simulink model "PID_differential_drive_robot"  (R2023b)
settings: Solver=VariableStepAuto  StartTime=0.0  StopTime=20  RelTol=1e-3
settings Model: Creator=patel  LastModifiedBy=patel

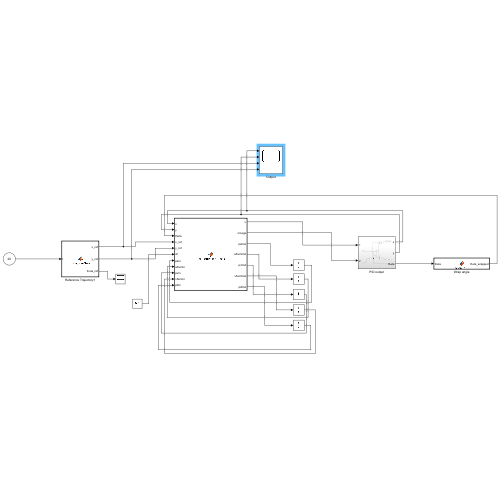
[thumbnail: Simulink's stored preview of the top-level diagram]
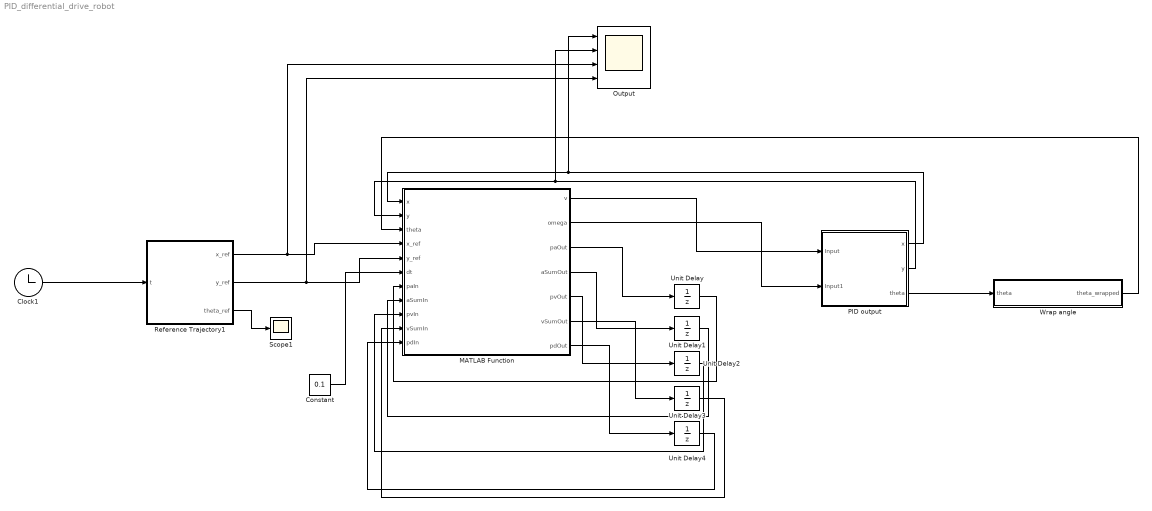
== system PID_differential_drive_robot ==
  Clock1 : Clock
      settings: Decimation=20
  Constant : Constant  Value=0.1
  MATLAB Function : MATLAB Function  TreatAsAtomicUnit=on
  Output : Scope  NumInputPorts=4
  PID output : Subsystem
  Reference Trajectory1 : MATLAB Function  TreatAsAtomicUnit=on
  Scope1 : Scope
  Unit Delay{,1..4} (5 alike) : UnitDelay  SampleTime=-1  HasFrameUpgradeWarning=on
  Wrap angle : MATLAB Function  TreatAsAtomicUnit=on
  wires:
  Clock1/1 -> Reference Trajectory1/1(t)
  Reference Trajectory1/1(x_ref) -> Output/3, MATLAB Function/4(x_ref)
  Reference Trajectory1/2(y_ref) -> Output/4, MATLAB Function/5(y_ref)
  Reference Trajectory1/3(theta_ref) -> Scope1/1
  MATLAB Function/1(v) -> PID output/1(Input)
  MATLAB Function/2(omega) -> PID output/2(Input1)
  PID output/3(theta) -> Wrap angle/1(theta)
  PID output/1(x) -> Output/1, MATLAB Function/1(x)
  PID output/2(y) -> Output/2, MATLAB Function/2(y)
  Wrap angle/1(theta_wrapped) -> MATLAB Function/3(theta)
  Constant/1 -> MATLAB Function/6(dt)
  MATLAB Function/3(paOut) -> Unit Delay/1
  Unit Delay/1 -> MATLAB Function/7(paIn)
  MATLAB Function/4(aSumOut) -> Unit Delay1/1
  Unit Delay1/1 -> MATLAB Function/8(aSumIn)
  MATLAB Function/5(pvOut) -> Unit Delay2/1
  Unit Delay2/1 -> MATLAB Function/9(pvIn)
  MATLAB Function/6(vSumOut) -> Unit Delay3/1
  Unit Delay3/1 -> MATLAB Function/10(vSumIn)
  MATLAB Function/7(pdOut) -> Unit Delay4/1
  Unit Delay4/1 -> MATLAB Function/11(pdIn)

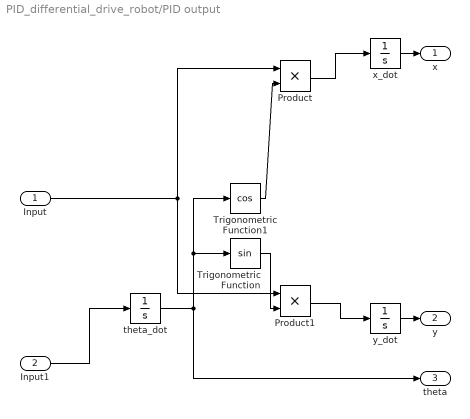
== system PID_differential_drive_robot/PID output ==
  Input : Inport
  Input1 : Inport  Port=2
  Product : Product
  Product1 : Product
  Trigonometric Function : Trigonometry
  Trigonometric Function1 : Trigonometry  Operator=cos
  theta_dot : Integrator
  x_dot : Integrator
  y_dot : Integrator
  x : Outport
  y : Outport  Port=2
  theta : Outport  Port=3
  wires:
  theta_dot/1 -> theta/1, Trigonometric Function1/1, Trigonometric Function/1
  Product/1 -> x_dot/1
  Input1/1 -> theta_dot/1
  Trigonometric Function1/1 -> Product/2
  Input/1 -> Product1/1, Product/1
  Trigonometric Function/1 -> Product1/2
  Product1/1 -> y_dot/1
  x_dot/1 -> x/1
  y_dot/1 -> y/1

== matlab function PID_differential_drive_robot/Wrap angle ==
  data: theta input; theta_wrapped output
function theta_wrapped = wrapToPi(theta)
    theta_wrapped = mod(theta + pi, 2*pi) - pi;
end

== matlab function PID_differential_drive_robot/MATLAB Function ==
  data: x input; v output; y input; theta input; x_ref input; y_ref input; dt input; paIn input; aSumIn input; pvIn input; vSumIn input; pdIn input; omega output; paOut output; aSumOut output; pvOut output; vSumOut output; pdOut output
function [v, omega, paOut, aSumOut, pvOut, vSumOut, pdOut] = pid_controller_block(x, y, theta, x_ref, y_ref, dt, paIn, aSumIn, pvIn, vSumIn, pdIn)
%#codegen
robotState = [x; y; theta];
targetPoint = [x_ref; y_ref];
[v, omega, paOut, aSumOut, pvOut, vSumOut, pdOut] = PIDController(robotState, targetPoint, dt, paIn, aSumIn, pvIn, vSumIn, pdIn);

    function [v, omega, prevAngleError, angleErrorSum, prevVError, vErrorSum, prevDistance] = PIDController(robotState, targetPoint, dt, prevAngleError, angleErrorSum, prevVError, vErrorSum, prevDistance)
    % Unpack robot state
    x = robotState(1);
    y = robotState(2);
    theta = robotState(3);

    x_target = targetPoint(1);
    y_target = targetPoint(2);

    % Desired forward velocity
    v_desired = 5.0;

    %% --- Angular control (omega) ---
    angle_to_target = atan2(y_target - y, x_target - x);
    angle_error = atan2(sin(angle_to_target - theta), cos(angle_to_target - theta));
    angle_error_deriv = (angle_error - prevAngleError) / dt;
    angleErrorSum = angleErrorSum + angle_error * dt;
    angleErrorSum = min(max(angleErrorSum, -1.0), 1.0); % Anti-windup
    prevAngleError = angle_error;

    % PID gains for angular velocity
    kp_omega = 2.0;
    ki_omega = 1.0;
    kd_omega = 0.6;
    omega = kp_omega * angle_error + ki_omega * angleErrorSum + kd_omega * angle_error_deriv;
    omega = min(max(omega, -pi), pi);

    %% --- Linear velocity control ---
    dist_to_target = sqrt((x_target - x)^2 + (y_target - y)^2);
    v_current = (prevDistance - dist_to_target) / dt;
    prevDistance = dist_to_target;

    v_error = v_desired - v_current;
    v_error_deriv = (v_error - prevVError) / dt;
    vErrorSum = vErrorSum + v_error * dt;
    vErrorSum = min(max(vErrorSum, -2.0), 2.0); % Anti-windup
    prevVError = v_error;

    % PID gains for linear velocity
    kp_v = 1.0;
    ki_v = 0.5;
    kd_v = 0.2;
    v = kp_v * v_error + ki_v * vErrorSum + kd_v * v_error_deriv;

    % Reduce speed when not aligned with target
    v = v * cos(angle_error);

    % Clamp final velocity
    v = min(max(v, 0.2), 5.0);
end
    
end

== matlab function PID_differential_drive_robot/Reference Trajectory1 ==
  data: t input; x_ref output; y_ref output; theta_ref output
function [x_ref, y_ref, theta_ref] = trajectoryGen(t)
    radius = 5;
    omega_ref = 0.2;
    x_ref = radius * cos(omega_ref * t);
    y_ref = radius * sin(omega_ref * t);
    theta_ref = omega_ref * t + pi/2;
end
